simulink model "stanleypathtracking"  (R2025a)
settings: Solver=ode45  StartTime=0.0  StopTime=240  MaxStep=1  RelTol=1e-3
libraries: drivinglib x2, simulink_extras x1, matrix_library x1, drivingvehiclecontroller x1
settings Model: Creator=ockap  LastModifiedBy=tethracross
settings RTWCC: GPUComputeCapability=3.5

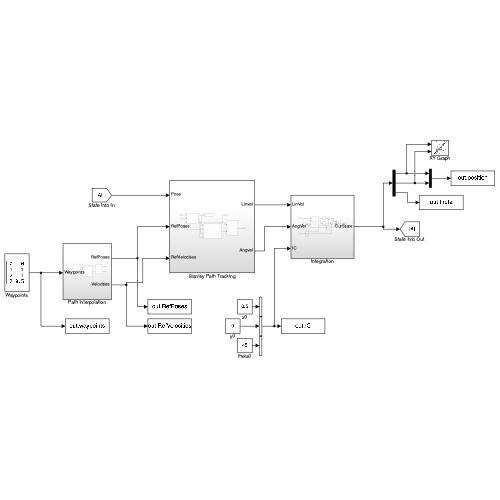
[thumbnail: Simulink's stored preview of the top-level diagram]
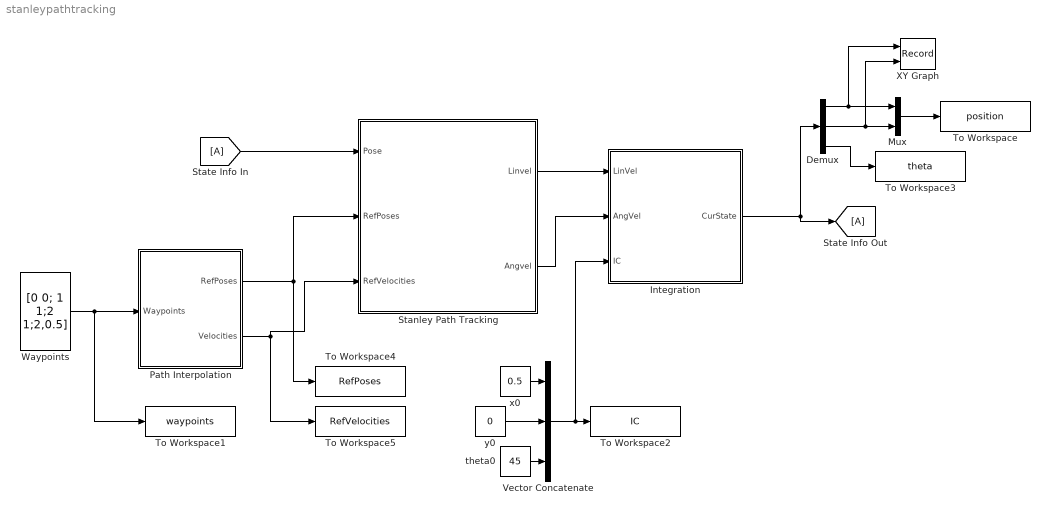
== system stanleypathtracking ==
  Demux : Demux  Outputs=3
  Integration : Subsystem
  Mux : Mux  Inputs=2
  Path Interpolation : Subsystem
  Stanley Path Tracking : Subsystem
  State Info In : From
  State Info Out : Goto
  To Workspace : ToWorkspace  VariableName=position  SaveFormat=Timeseries  SampleTime=-1
  To Workspace1 : ToWorkspace  VariableName=waypoints  SampleTime=-1
      settings: Save2DSignal=2-D array (concatenate along first dimension)
  To Workspace2 : ToWorkspace  VariableName=IC  SampleTime=-1
      settings: Save2DSignal=2-D array (concatenate along first dimension)
  To Workspace3 : ToWorkspace  VariableName=theta  SaveFormat=Timeseries  SampleTime=-1
  To Workspace4 : ToWorkspace  VariableName=RefPoses  SampleTime=-1
      settings: Save2DSignal=2-D array (concatenate along first dimension)
  To Workspace5 : ToWorkspace  VariableName=RefVelocities  SampleTime=-1
      settings: Save2DSignal=2-D array (concatenate along first dimension)
  Vector Concatenate : Concatenate  NumInputs=3
  Waypoints : Constant  Value=[0 0; 1 1;2 1;2,0.5]  VectorParams1D=off  SampleTime=-1
  XY Graph : Record  NumPorts=2.0  FileSettingsInternal="{\"entries\":[{\"content\":{\"excelSettings\":{\"content\":{},\"type\":\"Streamout.ExcelSettings\"},\"parquetSettings\":{\"content\":{},\"type\":\"Streamout.ParquetSettings\"}},\"type\":\"Streamout.FileSettingStorage\",\"uuid\":\"\"}],\"packageUris\":[\"http:\\/\\/schema.mathworks.com\\/mf0\\/streamout_blocks\\/R2020a\"],\"version\":\"1.0\"}"  FrameSettings=[0, 0]  Layout=[1 1]  SignalsInternal="{\"entries\":[{\"content\":{\"signals\":[{\"content\":{\"blockPath\":[],\"dimensions\":[1,1],\"domain\":\"\",\"lineColor\":\"#a2142f\",\"plots\":[ 1 ],\"port\":1,\"signalID\":1,\"signalName\":\"Demux:1\"},\"type\":\"RecordBlkView.Signal\",\"uuid\":\"\"},{\"content\":{\"blockPath\":[],\"dimensions\":[1,1],\"domain\":\"\",\"lineColor\":\"#139fff\",\"plots\":[ 1 ],\"port\":2,\"signalID\":2,\"signalName\":\"Demux:2\"},\"type\":\"RecordBlkView.Signal\",\"uuid\":\"\"}]},\"type\":\"RecordBlkView.InputSignals\",\"uuid\":\"\"}],\"packageUris\":[\"http:\\/\\/schema.mathworks.com\\/mf0\\/streamout_blocks\\/R2020a\"],\"version\":\"1.0\"}"  VisualizationBindings="{\"xyplotplugin\":{\"info\":[{\"series\":[{\"bindingParametersList\":[{\"parameter\":\"X-Axis\",\"signalID\":1,\"signalName\":\"Demux:1\"},{\"parameter\":\"Y-Axis\",\"signalID\":2,\"signalName\":\"Demux:2\"}],\"seriesID\":0}],\"subplotID\":1}]}}"  CompatibilityTag=XY
  theta0 : Constant  Value=45
  x0 : Constant  Value=0.5
  y0 : Constant  Value=0
  wires:
  Waypoints/1 -> Path Interpolation/1(Waypoints), To Workspace1/1
  Mux/1 -> To Workspace/1
  Demux/1 -> XY Graph/1, Mux/1
  Demux/2 -> XY Graph/2, Mux/2
  Demux/3 -> To Workspace3/1
  Stanley Path Tracking/1(Linvel) -> Integration/1(LinVel)
  Stanley Path Tracking/2(Angvel) -> Integration/2(AngVel)
  Path Interpolation/2(Velocities) -> To Workspace5/1, Stanley Path Tracking/3(RefVelocities)
  Path Interpolation/1(RefPoses) -> Stanley Path Tracking/2(RefPoses), To Workspace4/1
  Vector Concatenate/1 -> Integration/3(IC), To Workspace2/1
  theta0/1 -> Vector Concatenate/3
  x0/1 -> Vector Concatenate/1
  y0/1 -> Vector Concatenate/2
  Integration/1(CurState) -> State Info Out/1, Demux/1
  State Info In/1 -> Stanley Path Tracking/1(Pose)

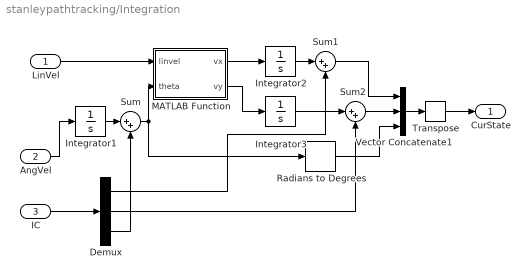
== system stanleypathtracking/Integration ==
  LinVel : Inport
  AngVel : Inport  Port=2
  IC : Inport  Port=3
  Demux : Demux  Outputs=3
  Integrator1 : Integrator
  Integrator2 : Integrator
  Integrator3 : Integrator
  MATLAB Function : MATLAB Function  TreatAsAtomicUnit=on
  Radians to Degrees : simulink_extras/Transformations/Radians to Degrees
  Sum : Sum  Inputs=|++
  Sum1 : Sum  Inputs=|++
  Sum2 : Sum  Inputs=|++
  Transpose : matrix_library/Transpose
  Vector Concatenate1 : Concatenate  NumInputs=3
  CurState : Outport
  wires:
  MATLAB Function/1(vx) -> Integrator2/1
  MATLAB Function/2(vy) -> Integrator3/1
  AngVel/1 -> Integrator1/1
  LinVel/1 -> MATLAB Function/1(linvel)
  Vector Concatenate1/1 -> Transpose/1
  Radians to Degrees/1 -> Vector Concatenate1/3
  Transpose/1 -> CurState/1
  Integrator1/1 -> Sum/1
  Sum/1 -> Radians to Degrees/1, MATLAB Function/2(theta)
  Demux/3 -> Sum/2
  Integrator2/1 -> Sum1/1
  Demux/1 -> Sum1/2
  Demux/2 -> Sum2/2
  Integrator3/1 -> Sum2/1
  Sum2/1 -> Vector Concatenate1/2
  Sum1/1 -> Vector Concatenate1/1
  IC/1 -> Demux/1

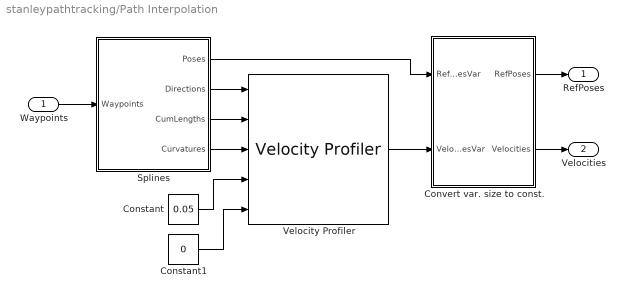
== system stanleypathtracking/Path Interpolation ==
  Waypoints : Inport
  Constant : Constant  Value=0.05
  Constant1 : Constant  Value=0
  Convert var. size to const. : MATLAB Function  TreatAsAtomicUnit=on
  Splines : Subsystem
  Velocity Profiler : drivinglib/Velocity Profiler  MaxLongitudinalAccel=0.05  MaxLongitudinalDecel=0.1  MaxSpeed=0.05  MaxLongitudinalJerk=0.1  MaxLateralAccel=0.1  ShowOptionalOutport=off  SampleTime=-1  SimulateUsing=Code generation
  RefPoses : Outport
  Velocities : Outport  Port=2
  wires:
  Waypoints/1 -> Splines/1(Waypoints)
  Splines/2(Directions) -> Velocity Profiler/1
  Splines/3(CumLengths) -> Velocity Profiler/2
  Splines/4(Curvatures) -> Velocity Profiler/3
  Splines/1(Poses) -> Convert var. size to const./1(RefPosesVar)
  Constant/1 -> Velocity Profiler/4
  Constant1/1 -> Velocity Profiler/5
  Convert var. size to const./1(RefPoses) -> RefPoses/1
  Velocity Profiler/1 -> Convert var. size to const./2(VelocitiesVar)
  Convert var. size to const./2(Velocities) -> Velocities/1

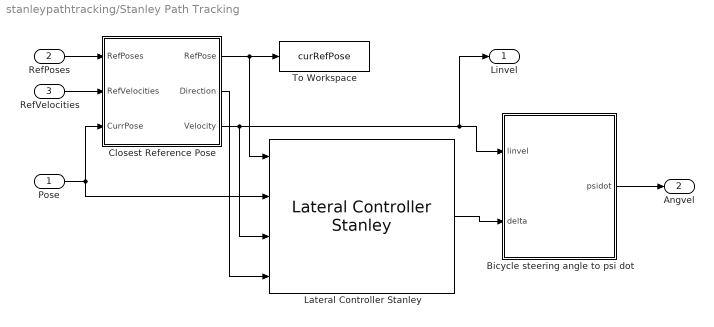
== system stanleypathtracking/Stanley Path Tracking ==
  Pose : Inport
  RefPoses : Inport  Port=2
  RefVelocities : Inport  Port=3
  Bicycle steering angle to psi dot : MATLAB Function  TreatAsAtomicUnit=on
  Closest Reference Pose : MATLAB Function  TreatAsAtomicUnit=on
  Lateral Controller Stanley : drivingvehiclecontroller/Lateral Controller Stanley  ModelType=Kinematic bicycle model  PositionGainF=5  PositionGainR=2.5  YawRateGain=0.2  DelayGain=0.2  VehicleMass=1575  Lf=1.2  Lr=1.6  TireStiffness=19000  Wheelbase=0.1  MaxSteeringAngle=35
  To Workspace : ToWorkspace  VariableName=curRefPose  SampleTime=-1
      settings: Save2DSignal=2-D array (concatenate along first dimension)
  Linvel : Outport
  Angvel : Outport  Port=2
  wires:
  Pose/1 -> Lateral Controller Stanley/2, Closest Reference Pose/3(CurrPose)
  Closest Reference Pose/2(Direction) -> Lateral Controller Stanley/4
  Closest Reference Pose/3(Velocity) -> Lateral Controller Stanley/3, Linvel/1, Bicycle steering angle to psi dot/1(linvel)
  Lateral Controller Stanley/1 -> Bicycle steering angle to psi dot/2(delta)
  Bicycle steering angle to psi dot/1(psidot) -> Angvel/1
  Closest Reference Pose/1(RefPose) -> To Workspace/1, Lateral Controller Stanley/1
  RefPoses/1 -> Closest Reference Pose/1(RefPoses)
  RefVelocities/1 -> Closest Reference Pose/2(RefVelocities)

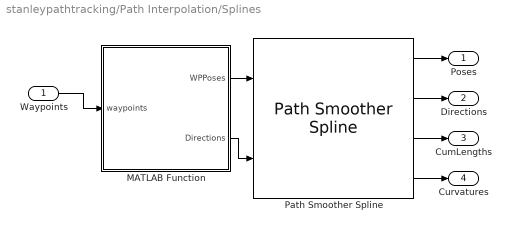
== system stanleypathtracking/Path Interpolation/Splines ==
  Waypoints : Inport
  MATLAB Function : MATLAB Function  TreatAsAtomicUnit=on
  Path Smoother Spline : drivinglib/Path Smoother Spline  NumSmoothPoses=100  MinSeparation=1e-3  SampleTime=1000  ShowOptionalOutports=on  SimulateUsing=Code generation
  Poses : Outport
      settings: VarSizeSig=Yes
  Directions : Outport  Port=2
  CumLengths : Outport  Port=3
  Curvatures : Outport  Port=4
  wires:
  Path Smoother Spline/2 -> Directions/1
  Path Smoother Spline/1 -> Poses/1
  MATLAB Function/1(WPPoses) -> Path Smoother Spline/1
  MATLAB Function/2(Directions) -> Path Smoother Spline/2
  Path Smoother Spline/3 -> CumLengths/1
  Path Smoother Spline/4 -> Curvatures/1
  Waypoints/1 -> MATLAB Function/1(waypoints)

== matlab function stanleypathtracking/Path Interpolation/Splines/MATLAB Function ==
  data: waypoints input; WPPoses output; Directions output
function [WPPoses,Directions] = waypoint2pose(waypoints)
    numpoints = height(waypoints);
    xpoints = waypoints(:,1);
    ypoints = waypoints(:,2);
    desiredheadings = zeros(numpoints,1);
    desiredheadings(1) = atan2d(ypoints(2)-ypoints(1),xpoints(2)-xpoints(1));
    desiredheadings(end) = atan2d(ypoints(numpoints)-ypoints(numpoints-1),xpoints(numpoints)-xpoints(numpoints-1));
    for n = 2:numpoints-1
        desiredheadings(n) = atan2d(ypoints(n+1)-ypoints(n-1),xpoints(n+1)-xpoints(n-1));
    end
    WPPoses = [waypoints desiredheadings];
    Directions = ones(size(desiredheadings));

== matlab function stanleypathtracking/Integration/MATLAB Function ==
  data: linvel input; vx output; theta input; vy output
function [vx,vy] = fcn(linvel,theta)
    vx = linvel*cos(theta);
    vy = linvel*sin(theta);
end

== matlab function stanleypathtracking/Stanley Path Tracking/Closest Reference Pose ==
  data: RefPoses input; RefPose output; Direction output; Velocity output; RefVelocities input; CurrPose input
function [RefPose,Direction,Velocity] = getrefpose(RefPoses,RefVelocities,CurrPose)
    waypoints = RefPoses(:,1:2);
    currcoord = CurrPose(1:2);
    wpdistances = waypoints - [currcoord(1)*ones(height(waypoints),1) currcoord(2)*ones(height(waypoints),1)];
    [~,refindex] = min(vecnorm(wpdistances,2,2));
    RefPose = RefPoses(refindex,1:3);
    Velocity = RefVelocities(refindex);
    Direction = 1;

== matlab function stanleypathtracking/Stanley Path Tracking/Bicycle steering angle to psi dot ==
  data: linvel input; delta input; psidot output
function psidot = bicyclesteertopsidot(linvel,delta)

psidot = (linvel * tand(delta)) / 0.1; %0.15 = bicycle length

== matlab function stanleypathtracking/Path Interpolation/Convert var. size to const. ==
  data: RefPosesVar input; RefPoses output; VelocitiesVar input; Velocities output
function [RefPoses,Velocities] = fcn(RefPosesVar,VelocitiesVar)
%need to convert to fixed size for some reason
RefPoses = RefPosesVar(1:100,1:3);
Velocities = VelocitiesVar(1:100);
